simulink model "robmovil_sim_15a"  (R2015a)
settings: Solver=ode45  StartTime=0.0  StopTime=T  RelTol=1e-3
undefined symbols (not defined in the file or in its folder): atan4, magnitude, x0, y0
libraries: simulink x1
settings Model: Creator=Juan Esteban  LastModifiedBy=Juan Esteban

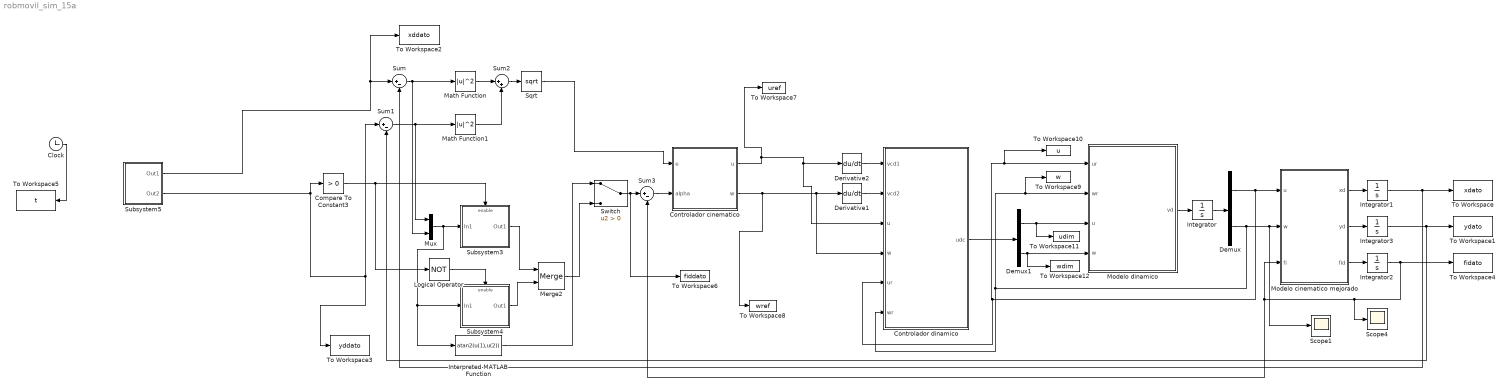
== system robmovil_sim_15a ==
  Clock : Clock
  Compare To Constant3 : simulink/Logic and Bit Operations/Compare To Constant  relop=>  const=0  OutDataTypeStr=boolean
  Controlador cinematico : MATLAB Function  TreatAsAtomicUnit=on
  Controlador dinamico : MATLAB Function  TreatAsAtomicUnit=on
  Demux : Demux  Outputs=2
  Demux1 : Demux  Outputs=2
  Derivative1 : Derivative
  Derivative2 : Derivative
  Integrator{,1..3} (4 alike) : Integrator
  Interpreted MATLAB Function : MATLABFcn  MATLABFcn=atan2(u(1),u(2))  OutputDimensions=1
  Logical Operator : Logic  Operator=NOT  AllPortsSameDT=off  OutDataTypeStr=boolean
  Math Function : Math  Operator=magnitude^2  SaturateOnIntegerOverflow=on
  Math Function1 : Math  Operator=magnitude^2  SaturateOnIntegerOverflow=on
  Merge2 : Merge
  Modelo cinematico mejorado : MATLAB Function  TreatAsAtomicUnit=on
  Modelo dinamico : MATLAB Function  TreatAsAtomicUnit=on
  Mux : Mux  Inputs=2
  Scope1 : Scope
      settings: YMin=-1.4672  YMax=1.93564
  Scope4 : Scope
      settings: YMin=-2.38151  YMax=5.71006  SaveName=ScopeData8
  Sqrt : Sqrt  SaturateOnIntegerOverflow=on
  Subsystem3 : Subsystem
  Subsystem4 : Subsystem
  Subsystem5 : Subsystem
  Sum : Sum  Inputs=|+-
  Sum1 : Sum  Inputs=|+-
  Sum2 : Sum  Inputs=|++
  Sum3 : Sum  Inputs=|+-
  Switch : Switch  Criteria=u2 > Threshold
  To Workspace : ToWorkspace  VariableName=xdato  SampleTime=-1
  To Workspace1 : ToWorkspace  VariableName=ydato  SampleTime=-1
  To Workspace10 : ToWorkspace  VariableName=u  SampleTime=-1
  To Workspace11 : ToWorkspace  VariableName=udim  SampleTime=-1
  To Workspace12 : ToWorkspace  VariableName=wdim  SampleTime=-1
  To Workspace2 : ToWorkspace  VariableName=xddato  SampleTime=-1
  To Workspace3 : ToWorkspace  VariableName=yddato  SampleTime=-1
  To Workspace4 : ToWorkspace  VariableName=fidato  SampleTime=-1
  To Workspace5 : ToWorkspace  VariableName=t  SampleTime=-1
  To Workspace6 : ToWorkspace  VariableName=fiddato  SampleTime=-1
  To Workspace7 : ToWorkspace  VariableName=uref  SampleTime=-1
  To Workspace8 : ToWorkspace  VariableName=wref  SampleTime=-1
  To Workspace9 : ToWorkspace  VariableName=w  SampleTime=-1
  wires:
  Math Function/1 -> Sum2/1
  Demux/1 -> Controlador dinamico/5(ur), To Workspace10/1, Modelo dinamico/1(ur), Modelo cinematico mejorado/1(u)
  Controlador dinamico/1(udc) -> Demux1/1
  Sum1/1 -> Mux/1, Math Function1/1
  Sum/1 -> Mux/2, Math Function/1
  Sum2/1 -> Sqrt/1
  Integrator2/1 -> Scope4/1, Modelo cinematico mejorado/3(fi), Sum3/2, To Workspace4/1
  Subsystem5/2(Out2) -> Sum1/1, To Workspace3/1, Compare To Constant3/1
  Integrator/1 -> Demux/1
  Modelo cinematico mejorado/2(yd) -> Integrator3/1
  Integrator3/1 -> To Workspace1/1, Sum1/2
  Modelo cinematico mejorado/1(xd) -> Integrator1/1
  Integrator1/1 -> Sum/2, To Workspace/1
  Subsystem5/1(Out1) -> To Workspace2/1, Sum/1
  Derivative1/1 -> Controlador dinamico/2(vcd2)
  Math Function1/1 -> Sum2/2
  Derivative2/1 -> Controlador dinamico/1(vcd1)
  Demux/2 -> To Workspace9/1, Modelo dinamico/2(wr), Controlador dinamico/6(wr), Scope1/1, Modelo cinematico mejorado/2(w)
  Modelo dinamico/1(vd) -> Integrator/1
  Modelo cinematico mejorado/3(fid) -> Integrator2/1
  Demux1/1 -> Modelo dinamico/3(u), To Workspace11/1
  Demux1/2 -> Modelo dinamico/4(w), To Workspace12/1
  Mux/1 -> Subsystem3/1(In1), Interpreted MATLAB Function/1, Subsystem4/1(In1)
  Subsystem3/1(Out1) -> Merge2/1
  Subsystem4/1(Out1) -> Merge2/2
  Logical Operator/1 -> Subsystem4/Enable
  Compare To Constant3/1 -> Logical Operator/1, Subsystem3/Enable
  Interpreted MATLAB Function/1 -> Switch/1
  Merge2/1 -> Switch/3
  Switch/1 -> To Workspace6/1, Sum3/1
  Sqrt/1 -> Controlador cinematico/1(e)
  Controlador cinematico/2(w) -> To Workspace8/1, Controlador dinamico/4(w), Derivative1/1
  Controlador cinematico/1(u) -> To Workspace7/1, Controlador dinamico/3(u), Derivative2/1
  Sum3/1 -> Controlador cinematico/2(alpha)
  Clock/1 -> To Workspace5/1

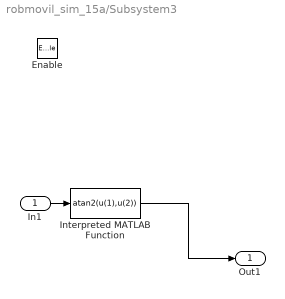
== system robmovil_sim_15a/Subsystem3 ==
  In1 : Inport
  Enable : EnablePort
  Interpreted MATLAB Function : MATLABFcn  MATLABFcn=atan2(u(1),u(2))  OutputDimensions=1
  Out1 : Outport
  wires:
  In1/1 -> Interpreted MATLAB Function/1
  Interpreted MATLAB Function/1 -> Out1/1

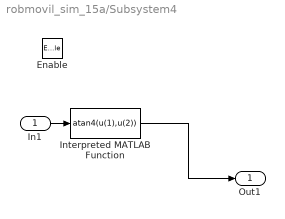
== system robmovil_sim_15a/Subsystem4 ==
  In1 : Inport
  Enable : EnablePort
  Interpreted MATLAB Function : MATLABFcn  MATLABFcn=atan4(u(1),u(2))  OutputDimensions=1
  Out1 : Outport
  wires:
  Interpreted MATLAB Function/1 -> Out1/1
  In1/1 -> Interpreted MATLAB Function/1

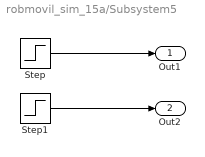
== system robmovil_sim_15a/Subsystem5 ==
  Step : Step  Time=0  After=x0  SampleTime=0
  Step1 : Step  Time=0  After=y0  SampleTime=0
  Out1 : Outport
  Out2 : Outport  Port=2
  wires:
  Step/1 -> Out1/1
  Step1/1 -> Out2/1

== matlab function robmovil_sim_15a/Modelo cinematico mejorado ==
  data: u input; w input; xd output; fi input; yd output; fid output
function [xd,yd,fid]= fcn(u,w,fi)
%#codegen
a=0.1;
xd=u*cos(fi)-a*w*sin(fi);
yd=u*sin(fi)-a*w*cos(fi);
fid=w;

== matlab function robmovil_sim_15a/Modelo dinamico ==
  data: ur input; wr input; u input; vd output; w input
function vd = fcn(ur,wr,u,w)
%#codegen
theta1=0.4072;
theta2=0.2937;
theta3=-0.0287;
theta4=0.9979;
theta5=-0.0004;
theta6=0.9865;
M=[theta1 0;0 theta2];
theta=[theta1 theta2 theta3 theta4 theta5 theta6]';
n=[0 0 -(wr^2) ur 0 0;0 0 0 0 wr*ur wr]*theta;
ud=[u;w];
vd=inv(M)*(ud-n);

== matlab function robmovil_sim_15a/Controlador dinamico ==
  data: vcd1 input; vcd2 input; u input; w input; ur input; wr input; udc output
function udc = fcn(vcd1,vcd2,u,w,ur,wr)
%#codegen
theta1=0.4072;
theta2=0.2937;
theta3=-0.0287;
theta4=0.9979;
theta5=-0.0004;
theta6=0.9865;
Qd=[1 0;0 1];
Kd=[1 0;0 1];
vcd=[vcd1;vcd2];
M=[theta1 0;0 theta2];
theta=[theta1 theta2 theta3 theta4 theta5 theta6]';
n=[0 0 -(wr^2) ur 0 0;0 0 0 0 wr*ur wr]*theta;
ve=[(u-ur);(w-wr)];
sigma=vcd+Qd*tanh(inv(Qd)*Kd*ve);
udc=M*sigma+n;

== matlab function robmovil_sim_15a/Controlador cinematico ==
  data: u output; e input; alpha input; w output
function [u,w] = fcn(e,alpha)
%#codegen
u=1*tanh(e)*cos(alpha);
w=alpha+tanh(e)/e*sin(alpha)*cos(alpha);
